simulink model "cos_and_cot_function"  (R2021a)
settings: Solver=VariableStepAuto  StartTime=0.0  StopTime=10.0  RelTol=1e-3
InitFcn:
  | w1=pi
  | w2 = 2*pi
  | A=6
  | B=4
settings Model: Creator=DELL  LastModifiedBy=DELL

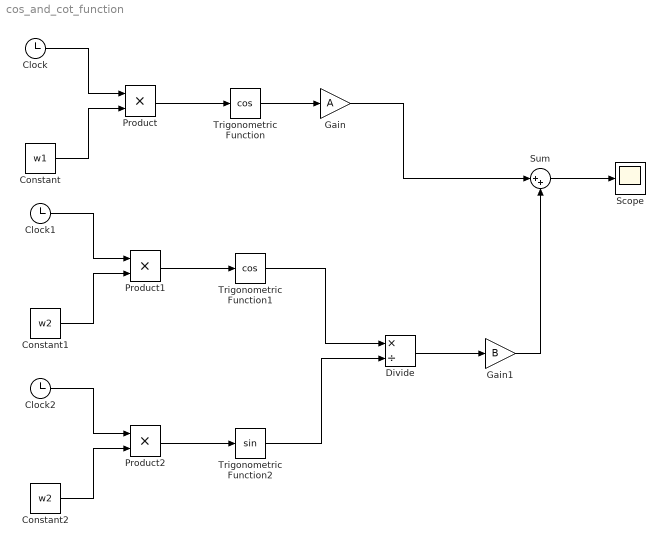
== system cos_and_cot_function ==
  Clock : Clock
  Clock1 : Clock
  Clock2 : Clock
  Constant : Constant  Value=w1
  Constant1 : Constant  Value=w2
  Constant2 : Constant  Value=w2
  Divide : Product  Inputs=*/
  Gain : Gain  Gain=A
  Gain1 : Gain  Gain=B
  Product : Product
  Product1 : Product
  Product2 : Product
  Scope : Scope
  Sum : Sum  Inputs=|++
  Trigonometric Function : Trigonometry  Operator=cos
  Trigonometric Function1 : Trigonometry  Operator=cos
  Trigonometric Function2 : Trigonometry
  wires:
  Constant/1 -> Product/2
  Clock/1 -> Product/1
  Product/1 -> Trigonometric Function/1
  Trigonometric Function/1 -> Gain/1
  Trigonometric Function1/1 -> Divide/1
  Product1/1 -> Trigonometric Function1/1
  Clock1/1 -> Product1/1
  Constant1/1 -> Product1/2
  Gain/1 -> Sum/1
  Sum/1 -> Scope/1
  Constant2/1 -> Product2/2
  Clock2/1 -> Product2/1
  Product2/1 -> Trigonometric Function2/1
  Trigonometric Function2/1 -> Divide/2
  Divide/1 -> Gain1/1
  Gain1/1 -> Sum/2
